simulink model "test"  (R2018a)
settings: Solver=VariableStepAuto  StartTime=0.0  StopTime=0  MaxStep=1e-3  RelTol=1e-3  AbsTol=1e-3
libraries: nesl_utility x57, pe_lib x52, fl_lib x43
Description:
  | Marine Full Electric Propulsion Power System
  | 
  | This example shows a representative marine half-ship electrical power system with
  | base load, hotel load, bow thrusters and electric propulsion.
  | 
  | The principal components of the system are:
  | *) 30 MVA Gas Turbine, Round Rotor Alternator
  | *) 5 MVA Diesel Generator, Salient Pole Alternator
  | *) 11.5 MVA Base Load
  | *) 6 MVA Switched Hotel Load
  | *) 20 MVA Average-Value Propulsion Rectifier
  | *) 1 MVA Direct Online Start, Squirrel Cage Bow Thrusters
  | 
  | The sequence of events during the simulation is:
  | *) 10 seconds - Hotel Load disconnected
  | *) 20 seconds - Propulsion begins ramping up
  | *) 30 seconds - Full power ahead
  | *) 40 seconds - Propulsion begins ramping down
  | *) 50 seconds - Bow Thrusters start up
  | *) 60 seconds - Hotel Load connected
  | 
  | To view full results, run the simulation, and enter at the MATLAB(R) command
  | prompt: sscexplore(pe_marine_electrical_system_simlog)
  | 
  | 
  | 
  | Copyright 2008-2016 The MathWorks, Inc.
settings Model: Creator=MathWorks  LastModifiedBy=giovannirenda
settings SolverCC: AutoScaleAbsTol=off  MaxConsecutiveMinStep=5  ZeroCrossAlgorithm=Adaptive
settings DataIOCC: LimitDataPoints=on  SaveFormat=Array
settings OptimizationCC: BlockReduction=off  BooleanDataType=off  LifeSpan=inf
settings DebuggingCC: SaveWithParameterizedLinksMsg=none  UnderspecifiedInitializationDetection=Classic  MergeDetectMultiDrivingBlocksExec=none  SignalResolutionControl=TryResolveAllWithWarning  AllowSymbolicDim=off  StrictBusMsg=ErrorOnBusTreatedAsVector  SFUnexpectedBacktrackingDiag=warning  SFNoUnconditionalDefaultTransitionDiag=warning  SFExecutionAtInitializationDiag=none
settings HardwareCC: ProdBitPerPointer=32  ProdBitPerSizeT=32  ProdBitPerPtrDiffT=32  ProdLargestAtomicFloat=None  ProdIntDivRoundTo=Undefined  ProdEndianess=Unspecified  ProdWordSize=32  ProdHWDeviceType=32-bit Generic  TargetBitPerLong=64  TargetBitPerPointer=64  TargetBitPerSizeT=64  TargetBitPerPtrDiffT=64  TargetLongLongMode=on  TargetIntDivRoundTo=Zero  TargetEndianess=LittleEndian  TargetWordSize=64  TargetHWDeviceType=MATLAB Host  ProdEqTarget=off
settings ModelReferenceCC: PropagateSignalLabelsOutOfModel=off
settings CodeAppCC: StateflowObjectComments=on
settings GRTTargetCC: TargetLangStandard=C89/C90 (ANSI)  GeneratePreprocessorConditionals=Disable all
settings ConfigComp: CovMetricSettings=dw  CovHtmlReporting=on  CovSaveCumulativeToWorkspaceVar=on  CovSaveSingleToWorkspaceVar=on  CovExternalEMLEnable=off  CovSFcnEnable=off
settings SimscapeCC: SimscapeNormalizeSystem=off  SimscapeLogType=local  SimscapeLogName=pe_marine_electrical_system_simlog  SimscapeLogLimitData=off

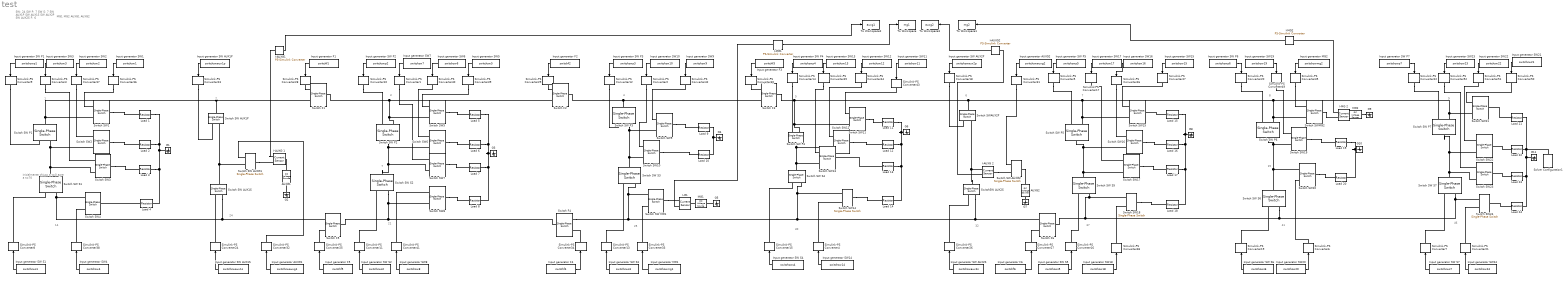
== system test ==
  note: MG1
      | MG2
      | AUXG1
      | AUXG2
  note: SW: 24
      | SW P: 7
      | SW S: 7
      | SW AUX1P
      | SW AUX1S
      | SW AUX2P
      | SW AUX2S
      | F: 6
  note: 41
  note: 32
  note: 6
  note: 4
  note: 2
  note: 24
  note: inizialmente
      | chiuso a t=0
      | apre a t=70
  note: 7
  note: 15
  note: 46
  note: 37
  note: 3
  note: 1
  note: 14
  note: 25
  note: 21
  note: 5
  note: 30
  note: 7
  note: 8
  note: 9
  AUXG1 : fl_lib/Electrical/Electrical Sources/DC Voltage Source  v0=5000 V
  AUXG2 : fl_lib/Electrical/Electrical Sources/DC Voltage Source  v0=5000 V
  G{1..11} (11 alike) : fl_lib/Electrical/Electrical Elements/Electrical Reference
  I-AUXG 1 : fl_lib/Electrical/Electrical Sensors/Current Sensor
  I-AUXG 2 : fl_lib/Electrical/Electrical Sensors/Current Sensor
  I-AUXG1 : nesl_utility/PS-Simulink Converter  PhysicalDomain=network_engine_domain  SubClassName=ps_output  LeftPortType=input  RightPortType=output  PseudoPeriodic=off  Frequencies=[]  Unit=A  AffineConversion=off
  I-AUXG2 : nesl_utility/PS-Simulink Converter  PhysicalDomain=network_engine_domain  SubClassName=ps_output  LeftPortType=input  RightPortType=output  PseudoPeriodic=off  Frequencies=[]  Unit=A  AffineConversion=off
  I-G1 : fl_lib/Electrical/Electrical Sensors/Current Sensor
  I-MG 2 : fl_lib/Electrical/Electrical Sensors/Current Sensor
  "I-MG1 " : nesl_utility/PS-Simulink Converter  PhysicalDomain=network_engine_domain  SubClassName=ps_output  LeftPortType=input  RightPortType=output  PseudoPeriodic=off  Frequencies=[]  Unit=A  AffineConversion=off
  "I-MG2 " : nesl_utility/PS-Simulink Converter  PhysicalDomain=network_engine_domain  SubClassName=ps_output  LeftPortType=input  RightPortType=output  PseudoPeriodic=off  Frequencies=[]  Unit=A  AffineConversion=off
  Input generator AUXG1 : FromWorkspace  VariableName=switchswauxg1  SampleTime=1
  Input generator AUXG2 : FromWorkspace  VariableName=switchswauxg2  SampleTime=1
  Input generator F1 : FromWorkspace  VariableName=switchf1  SampleTime=1
  Input generator F2 : FromWorkspace  VariableName=switchf2  SampleTime=1
  Input generator F3 : FromWorkspace  VariableName=switchf3  SampleTime=1
  Input generator F4 : FromWorkspace  VariableName=switchf4  SampleTime=1
  Input generator F5 : FromWorkspace  VariableName=switchf5  SampleTime=1
  Input generator F6 : FromWorkspace  VariableName=switchf6  SampleTime=1
  Input generator MG1 : FromWorkspace  VariableName=switchswmg1  SampleTime=1
  Input generator MG2 : FromWorkspace  VariableName=switchswmg2  SampleTime=1
  Input generator SW AUX1P : FromWorkspace  VariableName=switchswaux1p  SampleTime=1
  Input generator SW AUX1S : FromWorkspace  VariableName=switchswaux1s  SampleTime=1
  Input generator SW AUX2P : FromWorkspace  VariableName=switchswaux2p  SampleTime=1
  Input generator SW AUX2S : FromWorkspace  VariableName=switchswaux2s  SampleTime=1
  Input generator SW P1 : FromWorkspace  VariableName=switchswp1  SampleTime=1
  Input generator SW P2 : FromWorkspace  VariableName=switchswp2  SampleTime=1
  Input generator SW P3 : FromWorkspace  VariableName=switchswp3  SampleTime=1
  Input generator SW P4 : FromWorkspace  VariableName=switchswp4  SampleTime=1
  Input generator SW P5 : FromWorkspace  VariableName=switchswp5  SampleTime=1
  Input generator SW P6 : FromWorkspace  VariableName=switchswp6  SampleTime=1
  Input generator SW P7 : FromWorkspace  VariableName=switchswp7  SampleTime=1
  Input generator SW S1 : FromWorkspace  VariableName=switchsws1  SampleTime=1
  Input generator SW S2 : FromWorkspace  VariableName=switchsws2  SampleTime=1
  Input generator SW S3 : FromWorkspace  VariableName=switchsws3  SampleTime=1
  Input generator SW S4 : FromWorkspace  VariableName=switchsws4  SampleTime=1
  Input generator SW S5 : FromWorkspace  VariableName=switchsws5  SampleTime=1
  Input generator SW S6 : FromWorkspace  VariableName=switchsws6  SampleTime=1
  Input generator SW S7 : FromWorkspace  VariableName=switchsws7  SampleTime=1
  Input generator SW1 : FromWorkspace  VariableName=switchsw1  SampleTime=1
  Input generator SW10 : FromWorkspace  VariableName=switchsw10  SampleTime=1
  Input generator SW11 : FromWorkspace  VariableName=switchsw11  SampleTime=1
  Input generator SW12 : FromWorkspace  VariableName=switchsw12  SampleTime=1
  Input generator SW13 : FromWorkspace  VariableName=switchsw13  SampleTime=1
  Input generator SW14 : FromWorkspace  VariableName=switchsw14  SampleTime=1
  Input generator SW15 : FromWorkspace  VariableName=switchsw15  SampleTime=1
  Input generator SW16 : FromWorkspace  VariableName=switchsw16  SampleTime=1
  Input generator SW17 : FromWorkspace  VariableName=switchsw17  SampleTime=1
  Input generator SW18 : FromWorkspace  VariableName=switchsw18  SampleTime=1
  Input generator SW19 : FromWorkspace  VariableName=switchsw19  SampleTime=1
  Input generator SW2 : FromWorkspace  VariableName=switchsw2  SampleTime=1
  Input generator SW20 : FromWorkspace  VariableName=switchsw20  SampleTime=1
  Input generator SW21 : FromWorkspace  VariableName=switchsw21  SampleTime=1
  Input generator SW22 : FromWorkspace  VariableName=switchsw22  SampleTime=1
  Input generator SW23 : FromWorkspace  VariableName=switchsw23  SampleTime=1
  Input generator SW24 : FromWorkspace  VariableName=switchsw24  SampleTime=1
  Input generator SW3 : FromWorkspace  VariableName=switchsw3  SampleTime=1
  Input generator SW4 : FromWorkspace  VariableName=switchsw4  SampleTime=1
  Input generator SW5 : FromWorkspace  VariableName=switchsw5  SampleTime=1
  Input generator SW6 : FromWorkspace  VariableName=switchsw6  SampleTime=1
  Input generator SW7 : FromWorkspace  VariableName=switchsw7  SampleTime=1
  Input generator SW8 : FromWorkspace  VariableName=switchsw8  SampleTime=1
  Input generator SW9 : FromWorkspace  VariableName=switchsw9  SampleTime=1
  Load {1..2,4..6,8..9,11..12,14..16,18..19,21..22,24} (17 alike) : fl_lib/Electrical/Electrical Elements/Resistor  R=50 Ohm  i_specify=off  i_priority=None  i=0 A  i_nominal_specify=off  i_nominal_unit=A  i_nominal_value=1  v_specify=off  v_priority=None  v=0 V  v_nominal_specify=off  v_nominal_unit=V  v_nominal_value=1
  Load {3,7,10,13,17,20,23} (7 alike) : fl_lib/Electrical/Electrical Elements/Resistor  R=25 Ohm  i_specify=off  i_priority=None  i=0 A  i_nominal_specify=off  i_nominal_unit=A  i_nominal_value=1  v_specify=off  v_priority=None  v=0 V  v_nominal_specify=off  v_nominal_unit=V  v_nominal_value=1
  MG1 : fl_lib/Electrical/Electrical Sources/DC Voltage Source  v0=5000 V
  MG2 : fl_lib/Electrical/Electrical Sources/DC Voltage Source  v0=5000 V
  Simulink-PS Converter{1..52} (52 alike) : nesl_utility/Simulink-PS Converter  PhysicalDomain=network_engine_domain  SubClassName=ps_input  LeftPortType=input  RightPortType=output  PseudoPeriodic=off  Frequencies=[]  NoiseDistribution=none  NoiseParameters=[]  Unit=1  AffineConversion=off  FilteringAndDerivatives=zero  SimscapeFilterOrder=1  InputFilterTimeConstant=0.001  UdotUserProvided=1
  Solver Configuration1 : nesl_utility/Solver Configuration  PhysicalDomain=network_engine_domain  SubClassName=solver  LeftPortType=input  RightPortType=generic  Tones=[]  Harmonics=[]  SimulateNoise=off  Profile=off  UseLocalSampling=off  EnableSwitchedLinearOptims=on  FrequencyDomain=off  UseCCode=off  RelTol=0.001  AbsTol=1e-06  MinStep=1e-09  ToWorkspace=off  RevertToSquareIcSolve=off  NumHomotopyIterations=100  PhasorMode=off  PhasorModeNumHarmonics=1  DoDC=off  ResidualTolerance=1e-09  UseLocalSolver=off  LocalSolverChoice=NE_BACKWARD_EULER_ADVANCER  LocalSolverSampleTime=0.001  DoFixedCost=off  MaxNonlinIter=3  MaxModeIter=2  LinearAlgebra=Sparse  EquationFormulation=NE_TIME_EF  DelaysMemoryBudget=1024  AutomaticFiltering=on  FilteringTimeConstant=0.001
  Switch F{1..6} (6 alike) : pe_lib/Switches & Breakers/Fundamental Components/Single-Phase Switch  R_closed=0.001 Ohm  G_open=1e-6 1/Ohm  threshold=0 V
      settings: SourceProductName=Simscape Power Systems  SourceProductBaseCode=PS
  Switch SW AUX1P : pe_lib/Switches & Breakers/Fundamental Components/Single-Phase Switch  R_closed=0.001 Ohm  G_open=1e-6 1/Ohm  threshold=0 V
      settings: SourceProductName=Simscape Power Systems  SourceProductBaseCode=PS
  Switch SW AUX1S : pe_lib/Switches & Breakers/Fundamental Components/Single-Phase Switch  R_closed=0.001 Ohm  G_open=1e-6 1/Ohm  threshold=0 V
      settings: SourceProductName=Simscape Power Systems  SourceProductBaseCode=PS
  Switch SW AUXG1 : pe_lib/Switches & Breakers/Fundamental Components/Single-Phase Switch  R_closed=0.001 Ohm  G_open=1e-6 1/Ohm  threshold=0 V
      settings: SourceProductName=Simscape Power Systems  SourceProductBaseCode=PS
  Switch SW MG1 : pe_lib/Switches & Breakers/Fundamental Components/Single-Phase Switch  R_closed=0.001 Ohm  G_open=1e-6 1/Ohm  threshold=0 V
      settings: SourceProductName=Simscape Power Systems  SourceProductBaseCode=PS
  Switch SW P{1..7} (7 alike) : pe_lib/Switches & Breakers/Fundamental Components/Single-Phase Switch  R_closed=0.001 Ohm  G_open=1e-6 1/Ohm  threshold=0 V
      settings: SourceProductName=Simscape Power Systems  SourceProductBaseCode=PS
  Switch SW S{1..7} (7 alike) : pe_lib/Switches & Breakers/Fundamental Components/Single-Phase Switch  R_closed=0.001 Ohm  G_open=1e-6 1/Ohm  threshold=0 V
      settings: SourceProductName=Simscape Power Systems  SourceProductBaseCode=PS
  Switch SW-AUXG2 : pe_lib/Switches & Breakers/Fundamental Components/Single-Phase Switch  R_closed=0.001 Ohm  G_open=1e-6 1/Ohm  threshold=0 V
      settings: SourceProductName=Simscape Power Systems  SourceProductBaseCode=PS
  Switch SW{1..24} (24 alike) : pe_lib/Switches & Breakers/Fundamental Components/Single-Phase Switch  R_closed=0.001 Ohm  G_open=1e-6 1/Ohm  threshold=0 V
      settings: SourceProductName=Simscape Power Systems  SourceProductBaseCode=PS
  Switch SWAUX2P : pe_lib/Switches & Breakers/Fundamental Components/Single-Phase Switch  R_closed=0.001 Ohm  G_open=1e-6 1/Ohm  threshold=0 V
      settings: SourceProductName=Simscape Power Systems  SourceProductBaseCode=PS
  Switch SWMG2 : pe_lib/Switches & Breakers/Fundamental Components/Single-Phase Switch  R_closed=0.001 Ohm  G_open=1e-6 1/Ohm  threshold=0 V
      settings: SourceProductName=Simscape Power Systems  SourceProductBaseCode=PS
  SwitchSW AUX2S : pe_lib/Switches & Breakers/Fundamental Components/Single-Phase Switch  R_closed=0.001 Ohm  G_open=1e-6 1/Ohm  threshold=0 V
      settings: SourceProductName=Simscape Power Systems  SourceProductBaseCode=PS
  To Workspace : ToWorkspace  VariableName=mg1  SampleTime=1
      settings: Save2DSignal=2-D array (concatenate along first dimension)
  To Workspace1 : ToWorkspace  VariableName=mg2  SampleTime=1
      settings: Save2DSignal=2-D array (concatenate along first dimension)
  To Workspace2 : ToWorkspace  VariableName=auxg1  SampleTime=1
      settings: Save2DSignal=2-D array (concatenate along first dimension)
  To Workspace3 : ToWorkspace  VariableName=auxg2  SampleTime=1
      settings: Save2DSignal=2-D array (concatenate along first dimension)
  wires:
  Input generator SW P1/1 -> Simulink-PS Converter9/1
  Input generator SW S1/1 -> Simulink-PS Converter8/1
  Input generator SW3/1 -> Simulink-PS Converter3/1
  Input generator SW S2/1 -> Simulink-PS Converter11/1
  Input generator SW P2/1 -> Simulink-PS Converter10/1
  Input generator SW7/1 -> Simulink-PS Converter1/1
  Input generator SW S3/1 -> Simulink-PS Converter13/1
  Input generator SW P3/1 -> Simulink-PS Converter12/1
  Input generator SW10/1 -> Simulink-PS Converter2/1
  Input generator SW S4/1 -> Simulink-PS Converter15/1
  Input generator SW P4/1 -> Simulink-PS Converter14/1
  Input generator SW14/1 -> Simulink-PS Converter4/1
  Input generator SW S5/1 -> Simulink-PS Converter16/1
  Input generator SW P5/1 -> Simulink-PS Converter5/1
  Input generator SW17/1 -> Simulink-PS Converter17/1
  Input generator SW AUX2P/1 -> Simulink-PS Converter18/1
  Input generator SW P6/1 -> Simulink-PS Converter20/1
  Input generator SW S6/1 -> Simulink-PS Converter19/1
  Input generator SW20/1 -> Simulink-PS Converter6/1
  Input generator SW S7/1 -> Simulink-PS Converter7/1
  Input generator SW P7/1 -> Simulink-PS Converter22/1
  Input generator SW24/1 -> Simulink-PS Converter21/1
  Input generator SW AUX1P/1 -> Simulink-PS Converter23/1
  "I-MG1 "/1 -> To Workspace/1
  Input generator SW AUX1S/1 -> Simulink-PS Converter24/1
  Input generator SW AUX2S/1 -> Simulink-PS Converter26/1
  Input generator F1/1 -> Simulink-PS Converter28/1
  Input generator F2/1 -> Simulink-PS Converter29/1
  Input generator F3/1 -> Simulink-PS Converter30/1
  "I-MG2 "/1 -> To Workspace1/1
  I-AUXG2/1 -> To Workspace3/1
  I-AUXG1/1 -> To Workspace2/1
  Input generator AUXG2/1 -> Simulink-PS Converter31/1
  Input generator AUXG1/1 -> Simulink-PS Converter32/1
  Input generator MG1/1 -> Simulink-PS Converter33/1
  Input generator F4/1 -> Simulink-PS Converter34/1
  Input generator MG2/1 -> Simulink-PS Converter35/1
  Input generator F5/1 -> Simulink-PS Converter25/1
  Input generator F6/1 -> Simulink-PS Converter27/1
  Input generator SW1/1 -> Simulink-PS Converter36/1
  Input generator SW2/1 -> Simulink-PS Converter37/1
  Input generator SW4/1 -> Simulink-PS Converter38/1
  Input generator SW5/1 -> Simulink-PS Converter39/1
  Input generator SW6/1 -> Simulink-PS Converter40/1
  Input generator SW8/1 -> Simulink-PS Converter41/1
  Input generator SW9/1 -> Simulink-PS Converter42/1
  Input generator SW11/1 -> Simulink-PS Converter43/1
  Input generator SW12/1 -> Simulink-PS Converter44/1
  Input generator SW13/1 -> Simulink-PS Converter45/1
  Input generator SW16/1 -> Simulink-PS Converter46/1
  Input generator SW15/1 -> Simulink-PS Converter47/1
  Input generator SW18/1 -> Simulink-PS Converter48/1
  Input generator SW19/1 -> Simulink-PS Converter49/1
  Input generator SW21/1 -> Simulink-PS Converter50/1
  Input generator SW22/1 -> Simulink-PS Converter51/1
  Input generator SW23/1 -> Simulink-PS Converter52/1
  connections:
  Load 1/RConn1 -- G1/LConn1 -- Load 3/RConn1 -- Load 4/RConn1 -- Load 2/RConn1
  G2/LConn1 -- AUXG1/RConn1
  G5/LConn1 -- MG1/RConn1
  G7/LConn1 -- AUXG2/RConn1
  Switch SW S1/RConn1 -- Switch SW3/LConn2 -- Switch SW2/LConn2 -- Switch SW P1/LConn2
  Simulink-PS Converter9/RConn1 -- Switch SW P1/LConn1
  Simulink-PS Converter8/RConn1 -- Switch SW S1/LConn1
  Simulink-PS Converter3/RConn1 -- Switch SW3/LConn1
  Load 5/RConn1 -- G3/LConn1 -- Load 7/RConn1 -- Load 8/RConn1 -- Load 6/RConn1
  Switch SW S2/RConn1 -- Switch SW7/LConn2 -- Switch SW P2/RConn1 -- Switch SW6/LConn2
  Simulink-PS Converter1/RConn1 -- Switch SW7/LConn1
  Simulink-PS Converter10/RConn1 -- Switch SW P2/LConn1
  Simulink-PS Converter11/RConn1 -- Switch SW S2/LConn1
  Load 10/RConn1 -- Load 9/RConn1 -- G4/LConn1
  Simulink-PS Converter2/RConn1 -- Switch SW10/LConn1
  Simulink-PS Converter13/RConn1 -- Switch SW S3/LConn1
  Simulink-PS Converter12/RConn1 -- Switch SW P3/LConn1
  Switch SW P3/LConn2 -- Switch SW9/LConn2 -- Switch SW10/LConn2 -- Switch SW S3/RConn1
  Load 14/RConn1 -- G6/LConn1 -- Load 11/RConn1 -- Load 12/RConn1 -- Load 13/RConn1
  Switch SW S4/RConn1 -- Switch SW P4/RConn1 -- Switch SW12/LConn2 -- Switch SW13/LConn2
  Simulink-PS Converter4/RConn1 -- Switch SW14/LConn1
  Simulink-PS Converter15/RConn1 -- Switch SW S4/LConn1
  Simulink-PS Converter14/RConn1 -- Switch SW P4/LConn1
  Load 18/RConn1 -- Load 15/RConn1 -- G8/LConn1 -- Load 16/RConn1 -- Load 17/RConn1
  Switch SW S5/RConn1 -- Switch SW16/LConn2 -- Switch SW P5/RConn1 -- Switch SW17/LConn2
  Simulink-PS Converter5/RConn1 -- Switch SW P5/LConn1
  Simulink-PS Converter16/RConn1 -- Switch SW S5/LConn1
  Simulink-PS Converter18/RConn1 -- Switch SWAUX2P/LConn1
  Load 20/RConn1 -- Load 19/RConn1 -- G10/LConn1
  Switch SW P6/RConn1 -- Switch SW19/LConn2 -- Switch SW20/LConn2 -- Switch SW S6/RConn1
  Simulink-PS Converter19/RConn1 -- Switch SW S6/LConn1
  Simulink-PS Converter20/RConn1 -- Switch SW P6/LConn1
  Simulink-PS Converter6/RConn1 -- Switch SW20/LConn1
  Load 21/RConn1 -- Solver Configuration1/RConn1 -- G11/LConn1 -- Load 23/RConn1 -- Load 24/RConn1 -- Load 22/RConn1
  Switch SW S7/RConn1 -- Switch SW22/LConn2 -- Switch SW P7/RConn1 -- Switch SW23/LConn2
  Simulink-PS Converter7/RConn1 -- Switch SW S7/LConn1
  Simulink-PS Converter22/RConn1 -- Switch SW P7/LConn1
  Simulink-PS Converter23/RConn1 -- Switch SW AUX1P/LConn1
  Switch F5/LConn2 -- Switch SW AUX1S/LConn2 -- Switch SW S1/LConn2 -- Switch SW4/LConn2
  I-G1/RConn1 -- "I-MG1 "/LConn1
  Switch SW5/RConn1 -- Load 5/LConn1
  Switch SW6/RConn1 -- Load 6/LConn1
  Switch SW8/RConn1 -- Load 8/LConn1
  Switch SW AUX1S/RConn1 -- Switch SW AUXG1/LConn2 -- Switch SW AUX1P/LConn2
  Simulink-PS Converter24/RConn1 -- Switch SW AUX1S/LConn1
  SwitchSW AUX2S/RConn1 -- I-AUXG 2/RConn2 -- Switch SWAUX2P/LConn2
  Simulink-PS Converter26/RConn1 -- SwitchSW AUX2S/LConn1
  Switch SWMG2/LConn2 -- Switch SW P7/LConn2 -- Switch SW21/LConn2 -- Switch SW P5/LConn2 -- Switch SW15/LConn2 -- Switch SWAUX2P/RConn1 -- Switch SW P4/LConn2 -- Switch SW11/LConn2 -- Switch F3/RConn1 -- Switch SW P6/LConn2
  MG2/RConn1 -- G9/LConn1
  Switch SW AUX1P/RConn1 -- Switch F1/LConn2 -- Switch SW1/LConn2 -- Switch SW P1/RConn1
  Simulink-PS Converter28/RConn1 -- Switch F1/LConn1
  Simulink-PS Converter29/RConn1 -- Switch F2/LConn1
  Switch F2/LConn2 -- Switch SW5/LConn2 -- Switch SW P2/LConn2 -- Switch F1/RConn1
  Simulink-PS Converter30/RConn1 -- Switch F3/LConn1
  Switch SW P3/RConn1 -- Switch F3/LConn2 -- Switch F2/RConn1
  I-MG 2/RConn1 -- "I-MG2 "/LConn1
  I-MG 2/LConn1 -- MG2/LConn1
  Switch SW3/RConn1 -- Load 3/LConn1
  Switch SW2/RConn1 -- Load 2/LConn1
  Switch SW1/RConn1 -- Load 1/LConn1
  Switch SW14/RConn1 -- Load 14/LConn1
  Switch SW11/RConn1 -- Load 11/LConn1
  Switch SW12/RConn1 -- Load 12/LConn1
  Switch SW9/RConn1 -- Load 9/LConn1
  I-AUXG 2/RConn1 -- I-AUXG2/LConn1
  I-AUXG 1/RConn1 -- I-AUXG1/LConn1
  Switch SW16/RConn1 -- Load 16/LConn1
  Switch SW18/RConn1 -- Load 18/LConn1
  Switch SW19/RConn1 -- Load 19/LConn1
  Switch SW-AUXG2/RConn1 -- AUXG2/LConn1
  I-AUXG 2/LConn1 -- Switch SW-AUXG2/LConn2
  Simulink-PS Converter31/RConn1 -- Switch SW-AUXG2/LConn1
  Simulink-PS Converter32/RConn1 -- Switch SW AUXG1/LConn1
  Simulink-PS Converter33/RConn1 -- Switch SW MG1/LConn1
  Simulink-PS Converter34/RConn1 -- Switch F4/LConn1
  Switch SW S3/LConn2 -- Switch SW MG1/LConn2 -- Switch F6/LConn2 -- SwitchSW AUX2S/LConn2 -- Switch SW14/LConn2 -- Switch SW S4/LConn2 -- Switch F4/LConn2
  Switch SW AUXG1/RConn1 -- I-AUXG 1/RConn2
  AUXG1/LConn1 -- I-AUXG 1/LConn1
  Switch SWMG2/RConn1 -- I-MG 2/RConn2
  Simulink-PS Converter35/RConn1 -- Switch SWMG2/LConn1
  Switch F5/RConn1 -- Switch SW8/LConn2 -- Switch SW S2/LConn2 -- Switch F4/RConn1
  Simulink-PS Converter25/RConn1 -- Switch F5/LConn1
  Simulink-PS Converter27/RConn1 -- Switch F6/LConn1
  Switch SW S7/LConn2 -- Switch SW S6/LConn2 -- Switch SW18/LConn2 -- Switch SW S5/LConn2 -- Switch F6/RConn1 -- Switch SW24/LConn2
  Simulink-PS Converter36/RConn1 -- Switch SW1/LConn1
  Simulink-PS Converter37/RConn1 -- Switch SW2/LConn1
  Load 4/LConn1 -- Switch SW4/RConn1
  Simulink-PS Converter38/RConn1 -- Switch SW4/LConn1
  Simulink-PS Converter39/RConn1 -- Switch SW5/LConn1
  Switch SW7/RConn1 -- Load 7/LConn1
  Simulink-PS Converter40/RConn1 -- Switch SW6/LConn1
  Simulink-PS Converter41/RConn1 -- Switch SW8/LConn1
  Switch SW10/RConn1 -- Load 10/LConn1
  I-G1/LConn1 -- MG1/LConn1
  Switch SW MG1/RConn1 -- I-G1/RConn2
  Simulink-PS Converter42/RConn1 -- Switch SW9/LConn1
  Simulink-PS Converter43/RConn1 -- Switch SW11/LConn1
  Simulink-PS Converter44/RConn1 -- Switch SW12/LConn1
  Load 13/LConn1 -- Switch SW13/RConn1
  Simulink-PS Converter45/RConn1 -- Switch SW13/LConn1
  Switch SW17/RConn1 -- Load 17/LConn1
  Load 15/LConn1 -- Switch SW15/RConn1
  Switch SW15/LConn1 -- Simulink-PS Converter47/RConn1
  Simulink-PS Converter46/RConn1 -- Switch SW16/LConn1
  Switch SW17/LConn1 -- Simulink-PS Converter17/RConn1
  Switch SW18/LConn1 -- Simulink-PS Converter48/RConn1
  Switch SW20/RConn1 -- Load 20/LConn1
  Simulink-PS Converter49/RConn1 -- Switch SW19/LConn1
  Load 21/LConn1 -- Switch SW21/RConn1
  Load 23/LConn1 -- Switch SW23/RConn1
  Switch SW21/LConn1 -- Simulink-PS Converter50/RConn1
  Simulink-PS Converter52/RConn1 -- Switch SW23/LConn1
  Simulink-PS Converter51/RConn1 -- Switch SW22/LConn1
  Simulink-PS Converter21/RConn1 -- Switch SW24/LConn1
  Load 24/LConn1 -- Switch SW24/RConn1
  Load 22/LConn1 -- Switch SW22/RConn1
